simulink model "curiosity_i2c"  (R2024b)
settings: Solver=FixedStepDiscrete  StartTime=0.0  StopTime=inf  FixedStep=1e-3  RelTol=1e-3  EnableMultiTasking=on
undefined symbols (not defined in the file): A0, ADC, D10, D7, D8, D9, DiscIntNeverNeededParam, Max, MaxPer, ms, NumBits1, NumBits2, P1, P58, P59, Pin, Resol, s, Timer, us
libraries: MCHP_Blockset x18, simulink x15
(part 1 of 3)
settings Model: SimulationMode=external  ExtModeEnableFloating=off  ExtModeTrigDuration=20  Creator=I52209  LastModifiedBy=I52209
settings SolverCC: AlgebraicLoopSolver=TrustRegion
settings OptimizationCC: DefaultUnderspecifiedDataType=single  EnhancedBackFolding=on  BooleansAsBitfields=on  PassReuseOutputArgsAs=Individual arguments  ZeroExternalMemoryAtStartup=off  ZeroInternalMemoryAtStartup=off  OptimizeBlockOrder=speed  DifferentSizesBufferReuse=on  EfficientTunableParamExpr=on
settings DebuggingCC: MultiTaskDSMMsg=none  MultiTaskCondExecSysMsg=none  MultiTaskRateTransMsg=warning  ParameterTunabilityLossMsg=error  ArithmeticOperatorsInVariantConditions=warning
settings HardwareCC: ProdBitPerPointer=32  ProdBitPerSizeT=32  ProdBitPerPtrDiffT=32  ProdLargestAtomicInteger=Long  ProdWordSize=32  ProdLongLongMode=on  ProdHWDeviceType=Generic->Custom
settings ModelReferenceCC: ModelReferenceNumInstancesAllowed=Single
settings SFSimCC: MATLABDynamicMemAlloc=off  CustomCodeUndefinedFunction=UseInterfaceOnly
settings RTWCC: Description=Microchip Embedded Target dsPIC33A (real-time)  SystemTargetFile=MCHP_dsPIC33A_stf.tlc  TLCOptions="-aExtModeXCPClassicInterface=0  -aCreateExtModeTypes=1 -aExtModeXCPSimulationTimeInTicks=1"  TemplateMakefile=MCHP_dsPIC33A.tmf  GPUComputeCapability=3.5
settings CodeAppCC: ForceParamTrailComments=on  IgnoreCustomStorageClasses=off  MaxIdLength=255  OperatorAnnotations=on  SimulinkDataObjDesc=on  SFDataObjDesc=on  InsertBlockDesc=on
settings STFCustomTargetCC: TargetLibSuffix=_lib.a  TargetLangStandard=C99 (ISO)  MultiwordLength=256  CombineOutputUpdateFcns=on  CombineSignalStateStructs=on  ERTCustomFileBanners=on  SupportContinuousTime=off  RemoveResetFunc=on  MATLABClassNameForMDSCustomization=Simulink.SoftwareTarget.ERTCustomization  SystemTargetFile=MCHP_dsPIC33A_stf.tlc
settings ERTTargetCC: TargetLibSuffix=_lib.a  TargetLangStandard=C99 (ISO)  ParMdlRefBuildCompliant=off  CompOptLevelCompliant=off  ConcurrentExecutionCompliant=off  CombineSignalStateStructs=on  SupportNonInlinedSFcns=on  ModelStepFunctionPrototypeControlCompliant=off  CPPClassGenCompliant=off  UseToolchainInfoCompliant=off  ExtMode=on  ExtModeTransport=1  ExtModeStaticAlloc=on  ExtModeStaticAllocSize=2048  ExtModeMexFile=ext_xcp  ExtModeMexArgs=1 52 460800 './curiosity_i2c.X/curiosity_i2c.elf'  ExtModeIntrfLevel=Level2 - Open  InlinedParameterPlacement=Hierarchical  ERTSrcFileBannerTemplate=MCHP_dsPIC_code_template.cgt  ERTHdrFileBannerTemplate=MCHP_dsPIC_code_template.cgt  ERTDataSrcFileTemplate=MCHP_dsPIC_code_template.cgt  ERTDataHdrFileTemplate=MCHP_dsPIC_code_template.cgt  ERTCustomFileTemplate=MCHP_main.tlc  MaxLineWidth=110  DynamicArrayContainerType=coder::array

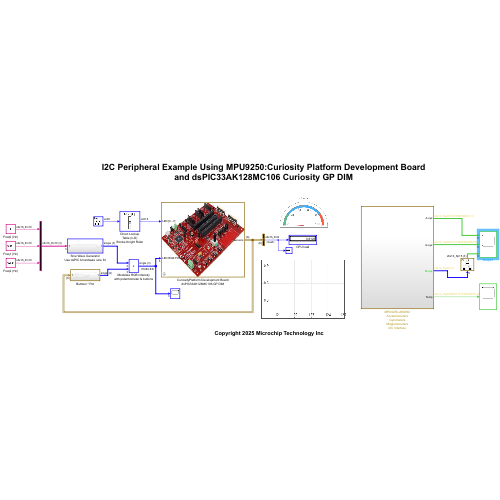
[thumbnail: Simulink's stored preview of the top-level diagram]
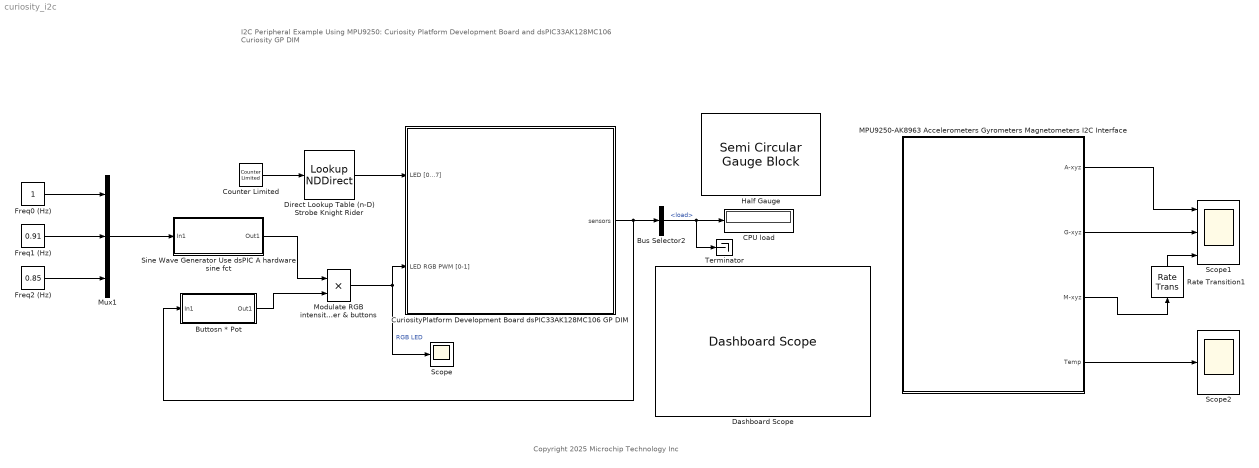
== system curiosity_i2c ==
  note: I2C Peripheral Example Using MPU9250: Curiosity Platform Development Board and dsPIC33AK128MC106 Curiosity GP DIM
  note: Copyright 2025 Microchip Technology Inc
  Bus Selector2 : BusSelector  OutputSignals=MCU.load
  Buttosn * Pot : Subsystem
  CPU load : Display
  Counter Limited : simulink/Sources/Counter Limited  uplimit=13  tsamp=0.05
  CuriosityPlatform Development Board dsPIC33AK128MC106 GP DIM : Subsystem
      mask Display: image('MCHP_i_Board_Curiosity_dsPICA.jpg')
  Dashboard Scope : DashboardScope  TimeSpan=5  Ymin=0  Ymax=1  LegendPosition=Hide  ScaleAtStop=off  TicksPosition=Inside
  Direct Lookup Table (n-D) Strobe Knight Rider : LookupNDDirect  NumberOfTableDimensions=1  Table=uint16(2.^[[0:7] [6:-1:1]] )  RemoveProtectionInput=on
  Freq0 (Hz) : Constant  OutDataTypeStr=fixdt(0,16,10)
  Freq1 (Hz) : Constant  Value=0.91  OutDataTypeStr=fixdt(0,16,10)
  Freq2 (Hz) : Constant  Value=0.85  OutDataTypeStr=fixdt(0,16,10)
  Half Gauge : SemiCircularGaugeBlock
  MPU9250-AK8963 Accelerometers Gyrometers Magnetometers I2C Interface : Subsystem
  Modulate RGB intensity with potentiometer & buttons : Product  OutDataTypeStr=single
  Mux1 : Mux  Inputs=3
  Rate Transition1 : RateTransition  Deterministic=off  OutPortSampleTimeOpt=Inherit
  Scope : Scope
  Scope1 : Scope  NumInputPorts=3
  Scope2 : Scope
  Sine Wave Generator Use dsPIC A hardware sine fct : Subsystem
  Terminator : Terminator
  wires:
  Buttosn * Pot/1(Out1) -> Modulate RGB intensity with potentiometer & buttons/2
  Bus Selector2/1 -> Terminator/1, CPU load/1  "<load>"
  Sine Wave Generator Use dsPIC A hardware sine fct/1(Out1) -> Modulate RGB intensity with potentiometer & buttons/1
  Mux1/1 -> Sine Wave Generator Use dsPIC A hardware sine fct/1(In1)
  Freq0 (Hz)/1 -> Mux1/1
  Freq1 (Hz)/1 -> Mux1/2
  Freq2 (Hz)/1 -> Mux1/3
  Direct Lookup Table (n-D) Strobe Knight Rider/1 -> CuriosityPlatform Development Board dsPIC33AK128MC106 GP DIM/1(LED [0...7])
  Modulate RGB intensity with potentiometer & buttons/1 -> CuriosityPlatform Development Board dsPIC33AK128MC106 GP DIM/2(LED RGB PWM [0-1]), Scope/1  "RGB LED"
  CuriosityPlatform Development Board dsPIC33AK128MC106 GP DIM/1(sensors) -> Buttosn * Pot/1(In1), Bus Selector2/1
  Counter Limited/1 -> Direct Lookup Table (n-D) Strobe Knight Rider/1
  MPU9250-AK8963 Accelerometers Gyrometers Magnetometers I2C Interface/3(M-xyz) -> Rate Transition1/1
  MPU9250-AK8963 Accelerometers Gyrometers Magnetometers I2C Interface/4(Temp) -> Scope2/1
  MPU9250-AK8963 Accelerometers Gyrometers Magnetometers I2C Interface/1(A-xyz) -> Scope1/1
  Rate Transition1/1 -> Scope1/3
  MPU9250-AK8963 Accelerometers Gyrometers Magnetometers I2C Interface/2(G-xyz) -> Scope1/2

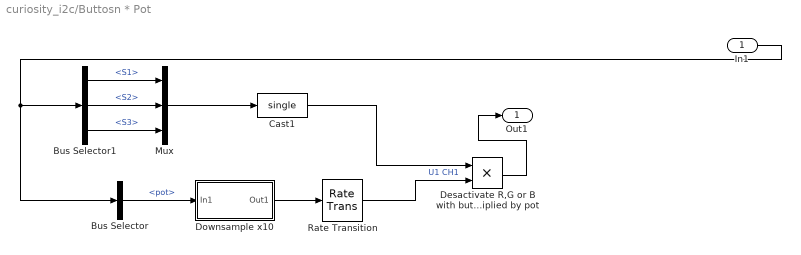
== system curiosity_i2c/Buttosn * Pot ==
  In1 : Inport
  Bus Selector : BusSelector  OutputSignals=ADC.pot
  Bus Selector1 : BusSelector  OutputSignals=BTN.S1,BTN.S2,BTN.S3
  Cast1 : DataTypeConversion  OutDataTypeStr=single  SaturateOnIntegerOverflow=off  RndMeth=Floor
  Desactivate R,G or B with buttons 1,2 or 3 multiplied by pot : Product  OutDataTypeStr=single
  Downsample x10 : Subsystem  mask{DownSample=10}
      mask prompts: DownSample "DownSample Factor"
  Mux : Mux  Inputs=3
  Rate Transition : RateTransition
  Out1 : Outport
  wires:
  Mux/1 -> Cast1/1
  Rate Transition/1 -> Desactivate R,G or B with buttons 1,2 or 3 multiplied by pot/2  "U1 CH1"
  In1/1 -> Bus Selector1/1, Bus Selector/1
  Bus Selector1/3 -> Mux/3  "<S3>"
  Downsample x10/1(Out1) -> Rate Transition/1
  Bus Selector/1 -> Downsample x10/1(In1)  "<pot>"
  Desactivate R,G or B with buttons 1,2 or 3 multiplied by pot/1 -> Out1/1
  Bus Selector1/1 -> Mux/1  "<S1>"
  Bus Selector1/2 -> Mux/2  "<S2>"
  Cast1/1 -> Desactivate R,G or B with buttons 1,2 or 3 multiplied by pot/1
